simulink model "Controller_Performance"  (R2022b)
settings: Solver=VariableStepAuto  StartTime=0.0  StopTime=10.0  RelTol=1e-3
undefined symbols (not defined in the file): den, K, num
settings Model: Creator=Akash  LastModifiedBy=Akash

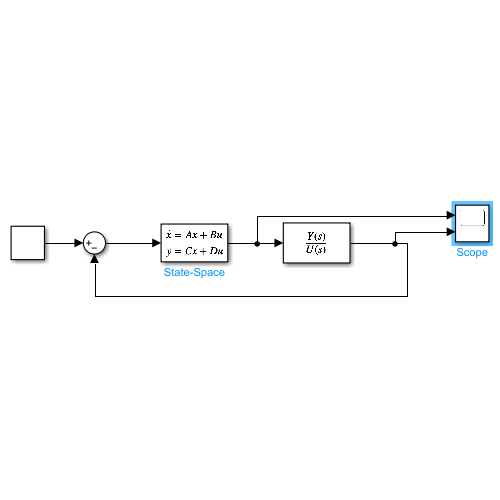
[thumbnail: Simulink's stored preview of the top-level diagram]
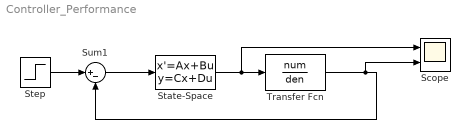
== system Controller_Performance ==
  Scope : Scope  NumInputPorts=2
  State-Space : StateSpace  A=K.A  B=K.B  C=K.C  D=K.D  InitialCondition=0
  Step : Step  SampleTime=0
  Sum1 : Sum  Inputs=|+-
  Transfer Fcn : TransferFcn  Numerator=num  Denominator=den
  wires:
  Transfer Fcn/1 -> Scope/2, Sum1/2
  Step/1 -> Sum1/1
  Sum1/1 -> State-Space/1
  State-Space/1 -> Scope/1, Transfer Fcn/1
